simulink model "simulink_02_nonlinear"  (R2025b)
settings: Solver=VariableStepAuto  StartTime=0.0  StopTime=23000  RelTol=1e-3
values from neighbouring files (symbols this model uses):
  mu = proximityP.mu    [CODE_42_02.m]
  n = proximityP.n    [CODE_42_02.m]
  proximityP = proximity_parameters()    [CODE_42_02.m]
  R0 = proximityP.R0    [CODE_42_02.m]
undefined symbols (not defined in the file or in its folder): K_1, ta, tb, tc, td
libraries: simulink x4
settings Model: Creator=palla  LastModifiedBy=palla

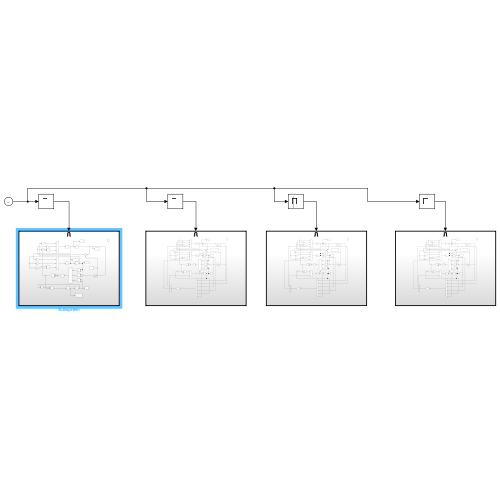
[thumbnail: Simulink's stored preview of the top-level diagram]
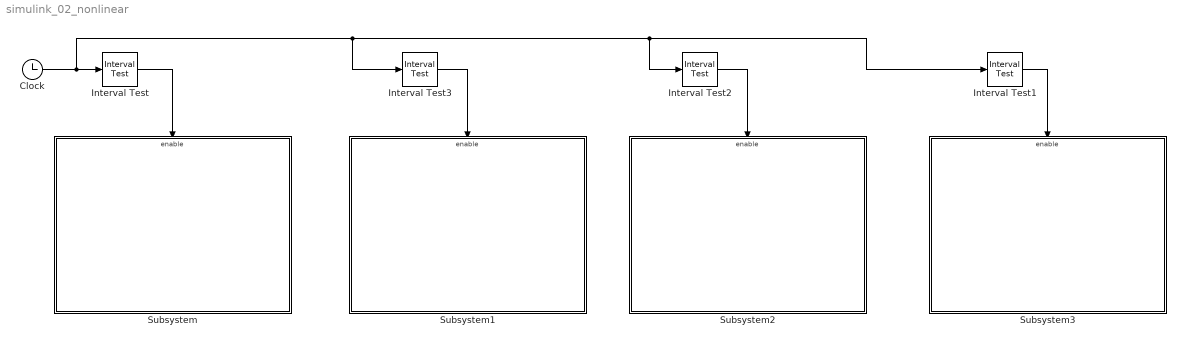
== system simulink_02_nonlinear ==
  Clock : Clock
  Interval Test : simulink/Logic and Bit Operations/Interval Test  IntervalClosedRight=on  uplimit=ta  IntervalClosedLeft=on  lowlimit=0  OutDataTypeStr=boolean
  Interval Test1 : simulink/Logic and Bit Operations/Interval Test  IntervalClosedRight=on  uplimit=td  IntervalClosedLeft=on  lowlimit=tc  OutDataTypeStr=boolean
  Interval Test2 : simulink/Logic and Bit Operations/Interval Test  IntervalClosedRight=on  uplimit=tc  IntervalClosedLeft=on  lowlimit=tb  OutDataTypeStr=boolean
  Interval Test3 : simulink/Logic and Bit Operations/Interval Test  IntervalClosedRight=on  uplimit=tb  IntervalClosedLeft=on  lowlimit=ta  OutDataTypeStr=boolean
  Subsystem : Subsystem
  Subsystem1 : Subsystem
  Subsystem2 : Subsystem
  Subsystem3 : Subsystem
  wires:
  Interval Test/1 -> Subsystem/Enable
  Clock/1 -> Interval Test1/1, Interval Test2/1, Interval Test3/1, Interval Test/1
  Interval Test3/1 -> Subsystem1/Enable
  Interval Test2/1 -> Subsystem2/Enable
  Interval Test1/1 -> Subsystem3/Enable

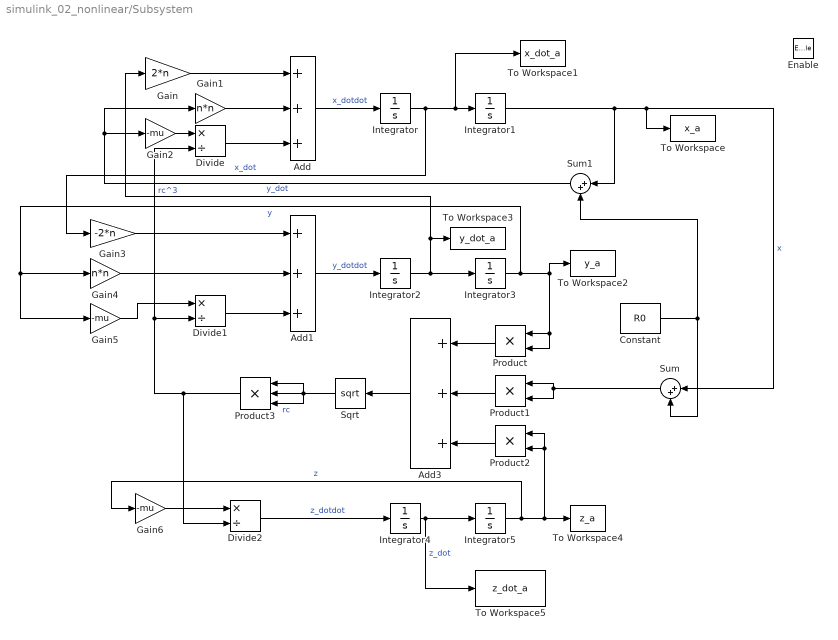
== system simulink_02_nonlinear/Subsystem ==
  Enable : EnablePort
  Add : Sum  Inputs=+++
  Add1 : Sum  Inputs=+++
  Add3 : Sum  Inputs=+++
  Constant : Constant  Value=R0
  Divide : Product  Inputs=*/
  Divide1 : Product  Inputs=*/
  Divide2 : Product  Inputs=*/
  Gain : Gain  Gain=2*n
  Gain1 : Gain  Gain=n*n
  Gain2 : Gain  Gain=-mu
  Gain3 : Gain  Gain=-2*n
  Gain4 : Gain  Gain=n*n
  Gain5 : Gain  Gain=-mu
  Gain6 : Gain  Gain=-mu
  Integrator : Integrator
  Integrator1 : Integrator  InitialCondition=0.1*1e3
  Integrator2 : Integrator  InitialCondition=-0.15*n*1e3
  Integrator3 : Integrator
  Integrator4 : Integrator
  Integrator5 : Integrator  InitialCondition=0.05*1e3
  Product : Product
  Product1 : Product
  Product2 : Product
  Product3 : Product  Inputs=3
  Sqrt : Sqrt
  Sum : Sum  Inputs=|++
  Sum1 : Sum  Inputs=|++
  To Workspace : ToWorkspace  VariableName=x_a  SampleTime=-1
  To Workspace1 : ToWorkspace  VariableName=x_dot_a  SampleTime=-1
  To Workspace2 : ToWorkspace  VariableName=y_a  SampleTime=-1
  To Workspace3 : ToWorkspace  VariableName=y_dot_a  SampleTime=-1
  To Workspace4 : ToWorkspace  VariableName=z_a  SampleTime=-1
  To Workspace5 : ToWorkspace  VariableName=z_dot_a  SampleTime=-1
  wires:
  Product2/1 -> Add3/3
  Divide2/1 -> Integrator4/1  "z_dotdot"
  Divide1/1 -> Add1/3
  Divide/1 -> Add/3
  Integrator5/1 -> Gain6/1, To Workspace4/1, Product2/1, Product2/2  "z"
  Add/1 -> Integrator/1  "x_dotdot"
  Gain4/1 -> Add1/2
  Gain6/1 -> Divide2/1
  Integrator2/1 -> Integrator3/1, To Workspace3/1, Gain/1  "y_dot"
  Integrator1/1 -> Sum1/1, To Workspace/1, Sum/1  "x"
  Integrator/1 -> Gain3/1, To Workspace1/1, Integrator1/1  "x_dot"
  Integrator4/1 -> To Workspace5/1, Integrator5/1  "z_dot"
  Integrator3/1 -> Gain5/1, Gain4/1, To Workspace2/1, Product/2, Product/1  "y"
  Product3/1 -> Divide1/2, Divide/2, Divide2/2  "rc^3"
  Constant/1 -> Sum1/2, Sum/2
  Add1/1 -> Integrator2/1  "y_dotdot"
  Sum1/1 -> Gain1/1, Gain2/1
  Sum/1 -> Product1/1, Product1/2
  Gain3/1 -> Add1/1
  Gain1/1 -> Add/2
  Product/1 -> Add3/1
  Product1/1 -> Add3/2
  Sqrt/1 -> Product3/3, Product3/1, Product3/2  "rc"
  Add3/1 -> Sqrt/1
  Gain/1 -> Add/1
  Gain2/1 -> Divide/1
  Gain5/1 -> Divide1/1

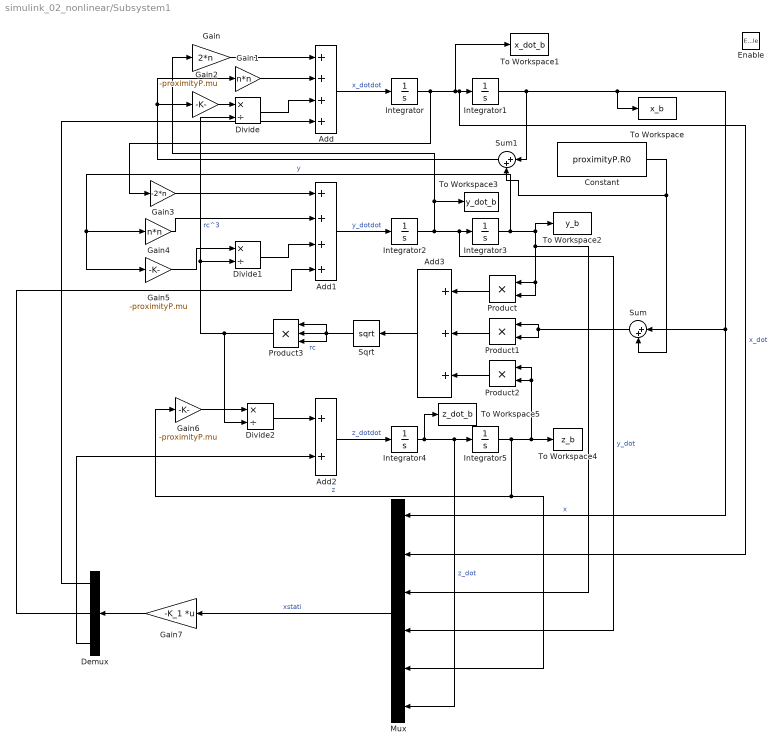
== system simulink_02_nonlinear/Subsystem1 ==
  Enable : EnablePort
  Add : Sum  Inputs=++++
  Add1 : Sum  Inputs=++++
  Add2 : Sum
  Add3 : Sum  Inputs=+++
  Constant : Constant  Value=proximityP.R0
  Demux : Demux  Outputs=3
  Divide : Product  Inputs=*/
  Divide1 : Product  Inputs=*/
  Divide2 : Product  Inputs=*/
  Gain : Gain  Gain=2*n
  Gain1 : Gain  Gain=n*n
  Gain2 : Gain  Gain=-proximityP.mu
  Gain3 : Gain  Gain=-2*n
  Gain4 : Gain  Gain=n*n
  Gain5 : Gain  Gain=-proximityP.mu
  Gain6 : Gain  Gain=-proximityP.mu
  Gain7 : Gain  Gain=-K_1  Multiplication=Matrix(K*u)
  Integrator{,1..5} (6 alike) : Integrator
  Mux : Mux  Inputs=6
  Product : Product
  Product1 : Product
  Product2 : Product
  Product3 : Product  Inputs=3
  Sqrt : Sqrt
  Sum : Sum  Inputs=|++
  Sum1 : Sum  Inputs=|++
  To Workspace : ToWorkspace  VariableName=x_b  SampleTime=-1
  To Workspace1 : ToWorkspace  VariableName=x_dot_b  SampleTime=-1
  To Workspace2 : ToWorkspace  VariableName=y_b  SampleTime=-1
  To Workspace3 : ToWorkspace  VariableName=y_dot_b  SampleTime=-1
  To Workspace4 : ToWorkspace  VariableName=z_b  SampleTime=-1
  To Workspace5 : ToWorkspace  VariableName=z_dot_b  SampleTime=-1
  wires:
  Product2/1 -> Add3/3
  Add2/1 -> Integrator4/1  "z_dotdot"
  Divide1/1 -> Add1/3
  Divide/1 -> Add/3
  Integrator5/1 -> Gain6/1, Mux/5, To Workspace4/1, Product2/1, Product2/2  "z"
  Add/1 -> Integrator/1  "x_dotdot"
  Demux/1 -> Add/4
  Gain4/1 -> Add1/2
  Gain6/1 -> Divide2/1
  Mux/1 -> Gain7/1  "xstati"
  Integrator2/1 -> Mux/4, Integrator3/1, Gain/1, To Workspace3/1  "y_dot"
  Integrator1/1 -> Sum1/1, To Workspace/1, Sum/1, Mux/1  "x"
  Integrator/1 -> Gain3/1, To Workspace1/1, Mux/2, Integrator1/1  "x_dot"
  Integrator4/1 -> Integrator5/1, Mux/6, To Workspace5/1  "z_dot"
  Integrator3/1 -> Gain5/1, Gain4/1, To Workspace2/1, Mux/3, Product/2, Product/1  "y"
  Product3/1 -> Divide1/2, Divide/2, Divide2/2  "rc^3"
  Constant/1 -> Sum1/2, Sum/2
  Add1/1 -> Integrator2/1  "y_dotdot"
  Sum1/1 -> Gain2/1, Gain1/1
  Sum/1 -> Product1/1, Product1/2
  Gain3/1 -> Add1/1
  Gain1/1 -> Add/2
  Product/1 -> Add3/1
  Gain7/1 -> Demux/1
  Product1/1 -> Add3/2
  Sqrt/1 -> Product3/3, Product3/1, Product3/2  "rc"
  Add3/1 -> Sqrt/1
  Gain/1 -> Add/1
  Demux/2 -> Add1/4
  Gain2/1 -> Divide/1
  Gain5/1 -> Divide1/1
  Divide2/1 -> Add2/1
  Demux/3 -> Add2/2

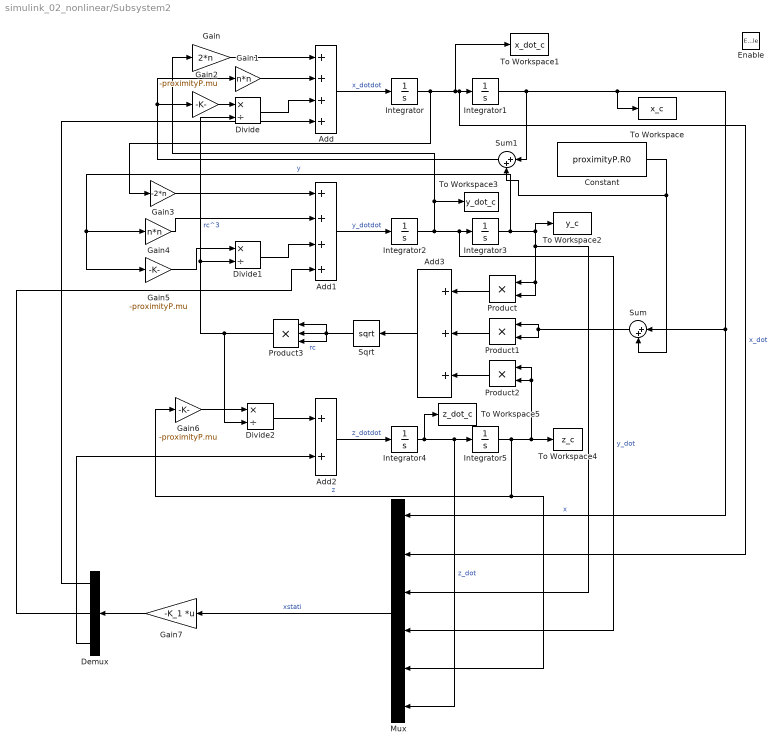
== system simulink_02_nonlinear/Subsystem2 ==
  Enable : EnablePort
  Add : Sum  Inputs=++++
  Add1 : Sum  Inputs=++++
  Add2 : Sum
  Add3 : Sum  Inputs=+++
  Constant : Constant  Value=proximityP.R0
  Demux : Demux  Outputs=3
  Divide : Product  Inputs=*/
  Divide1 : Product  Inputs=*/
  Divide2 : Product  Inputs=*/
  Gain : Gain  Gain=2*n
  Gain1 : Gain  Gain=n*n
  Gain2 : Gain  Gain=-proximityP.mu
  Gain3 : Gain  Gain=-2*n
  Gain4 : Gain  Gain=n*n
  Gain5 : Gain  Gain=-proximityP.mu
  Gain6 : Gain  Gain=-proximityP.mu
  Gain7 : Gain  Gain=-K_1  Multiplication=Matrix(K*u)
  Integrator{,1..5} (6 alike) : Integrator
  Mux : Mux  Inputs=6
  Product : Product
  Product1 : Product
  Product2 : Product
  Product3 : Product  Inputs=3
  Sqrt : Sqrt
  Sum : Sum  Inputs=|++
  Sum1 : Sum  Inputs=|++
  To Workspace : ToWorkspace  VariableName=x_c  SampleTime=-1
  To Workspace1 : ToWorkspace  VariableName=x_dot_c  SampleTime=-1
  To Workspace2 : ToWorkspace  VariableName=y_c  SampleTime=-1
  To Workspace3 : ToWorkspace  VariableName=y_dot_c  SampleTime=-1
  To Workspace4 : ToWorkspace  VariableName=z_c  SampleTime=-1
  To Workspace5 : ToWorkspace  VariableName=z_dot_c  SampleTime=-1
  wires:
  Product2/1 -> Add3/3
  Add2/1 -> Integrator4/1  "z_dotdot"
  Divide1/1 -> Add1/3
  Divide/1 -> Add/3
  Integrator5/1 -> Gain6/1, Mux/5, To Workspace4/1, Product2/1, Product2/2  "z"
  Add/1 -> Integrator/1  "x_dotdot"
  Demux/1 -> Add/4
  Gain4/1 -> Add1/2
  Gain6/1 -> Divide2/1
  Mux/1 -> Gain7/1  "xstati"
  Integrator2/1 -> Mux/4, Integrator3/1, Gain/1, To Workspace3/1  "y_dot"
  Integrator1/1 -> Sum1/1, To Workspace/1, Sum/1, Mux/1  "x"
  Integrator/1 -> Gain3/1, To Workspace1/1, Mux/2, Integrator1/1  "x_dot"
  Integrator4/1 -> Integrator5/1, Mux/6, To Workspace5/1  "z_dot"
  Integrator3/1 -> Gain5/1, Gain4/1, To Workspace2/1, Mux/3, Product/2, Product/1  "y"
  Product3/1 -> Divide1/2, Divide/2, Divide2/2  "rc^3"
  Constant/1 -> Sum1/2, Sum/2
  Add1/1 -> Integrator2/1  "y_dotdot"
  Sum1/1 -> Gain2/1, Gain1/1
  Sum/1 -> Product1/1, Product1/2
  Gain3/1 -> Add1/1
  Gain1/1 -> Add/2
  Product/1 -> Add3/1
  Gain7/1 -> Demux/1
  Product1/1 -> Add3/2
  Sqrt/1 -> Product3/3, Product3/1, Product3/2  "rc"
  Add3/1 -> Sqrt/1
  Gain/1 -> Add/1
  Demux/2 -> Add1/4
  Gain2/1 -> Divide/1
  Gain5/1 -> Divide1/1
  Divide2/1 -> Add2/1
  Demux/3 -> Add2/2

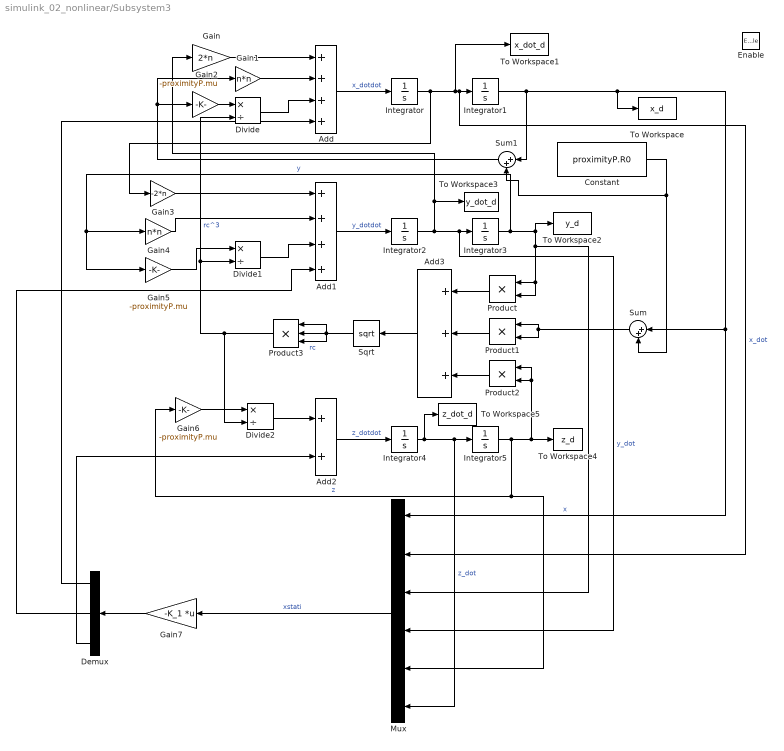
== system simulink_02_nonlinear/Subsystem3 ==
  Enable : EnablePort
  Add : Sum  Inputs=++++
  Add1 : Sum  Inputs=++++
  Add2 : Sum
  Add3 : Sum  Inputs=+++
  Constant : Constant  Value=proximityP.R0
  Demux : Demux  Outputs=3
  Divide : Product  Inputs=*/
  Divide1 : Product  Inputs=*/
  Divide2 : Product  Inputs=*/
  Gain : Gain  Gain=2*n
  Gain1 : Gain  Gain=n*n
  Gain2 : Gain  Gain=-proximityP.mu
  Gain3 : Gain  Gain=-2*n
  Gain4 : Gain  Gain=n*n
  Gain5 : Gain  Gain=-proximityP.mu
  Gain6 : Gain  Gain=-proximityP.mu
  Gain7 : Gain  Gain=-K_1  Multiplication=Matrix(K*u)
  Integrator{,1..5} (6 alike) : Integrator
  Mux : Mux  Inputs=6
  Product : Product
  Product1 : Product
  Product2 : Product
  Product3 : Product  Inputs=3
  Sqrt : Sqrt
  Sum : Sum  Inputs=|++
  Sum1 : Sum  Inputs=|++
  To Workspace : ToWorkspace  VariableName=x_d  SampleTime=-1
  To Workspace1 : ToWorkspace  VariableName=x_dot_d  SampleTime=-1
  To Workspace2 : ToWorkspace  VariableName=y_d  SampleTime=-1
  To Workspace3 : ToWorkspace  VariableName=y_dot_d  SampleTime=-1
  To Workspace4 : ToWorkspace  VariableName=z_d  SampleTime=-1
  To Workspace5 : ToWorkspace  VariableName=z_dot_d  SampleTime=-1
  wires:
  Product2/1 -> Add3/3
  Add2/1 -> Integrator4/1  "z_dotdot"
  Divide1/1 -> Add1/3
  Divide/1 -> Add/3
  Integrator5/1 -> Gain6/1, Mux/5, To Workspace4/1, Product2/1, Product2/2  "z"
  Add/1 -> Integrator/1  "x_dotdot"
  Demux/1 -> Add/4
  Gain4/1 -> Add1/2
  Gain6/1 -> Divide2/1
  Mux/1 -> Gain7/1  "xstati"
  Integrator2/1 -> Mux/4, Integrator3/1, Gain/1, To Workspace3/1  "y_dot"
  Integrator1/1 -> Sum1/1, To Workspace/1, Sum/1, Mux/1  "x"
  Integrator/1 -> Gain3/1, To Workspace1/1, Mux/2, Integrator1/1  "x_dot"
  Integrator4/1 -> Integrator5/1, Mux/6, To Workspace5/1  "z_dot"
  Integrator3/1 -> Gain5/1, Gain4/1, To Workspace2/1, Mux/3, Product/2, Product/1  "y"
  Product3/1 -> Divide1/2, Divide/2, Divide2/2  "rc^3"
  Constant/1 -> Sum1/2, Sum/2
  Add1/1 -> Integrator2/1  "y_dotdot"
  Sum1/1 -> Gain2/1, Gain1/1
  Sum/1 -> Product1/1, Product1/2
  Gain3/1 -> Add1/1
  Gain1/1 -> Add/2
  Product/1 -> Add3/1
  Gain7/1 -> Demux/1
  Product1/1 -> Add3/2
  Sqrt/1 -> Product3/3, Product3/1, Product3/2  "rc"
  Add3/1 -> Sqrt/1
  Gain/1 -> Add/1
  Demux/2 -> Add1/4
  Gain2/1 -> Divide/1
  Gain5/1 -> Divide1/1
  Divide2/1 -> Add2/1
  Demux/3 -> Add2/2
